simulink model "Differential_Equation"  (R2020b)
settings: Solver=VariableStepAuto  StartTime=0.0  StopTime=10.0  RelTol=1e-3
values from neighbouring files (symbols this model uses):
  a = 0.4    [data.mat]
  b = 0.5    [data.mat]
  c = 0.25    [data.mat]
settings Model: Creator=vijay jagtap  LastModifiedBy=vijay jagtap

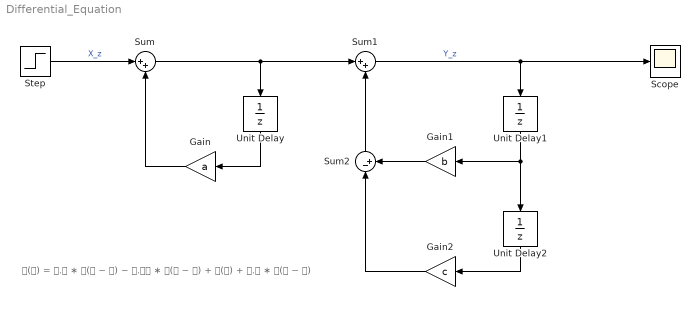
== system Differential_Equation ==
  note: 𝐲(𝐧) = 𝟎.𝟓 ∗ 𝐲(𝐧 − 𝟏) − 𝟎.𝟐𝟓 ∗ 𝐲(𝐧 − 𝟐) + 𝐱(𝐧) + 𝟎.𝟒 ∗ 𝐱(𝐧 − 𝟏)
  Gain : Gain  Gain=a
  Gain1 : Gain  Gain=b
  Gain2 : Gain  Gain=c
  Scope : Scope
  Step : Step  After=10  SampleTime=0
  Sum : Sum  Inputs=|++
  Sum1 : Sum  Inputs=|++
  Sum2 : Sum  Inputs=|-+
  Unit Delay : UnitDelay  SampleTime=-1  HasFrameUpgradeWarning=on
  Unit Delay1 : UnitDelay  SampleTime=-1  HasFrameUpgradeWarning=on
  Unit Delay2 : UnitDelay  SampleTime=-1  HasFrameUpgradeWarning=on
  wires:
  Sum2/1 -> Sum1/2
  Sum1/1 -> Scope/1, Unit Delay1/1  "Y_z"
  Gain1/1 -> Sum2/2
  Gain2/1 -> Sum2/1
  Unit Delay/1 -> Gain/1
  Gain/1 -> Sum/2
  Step/1 -> Sum/1  "X_z"
  Sum/1 -> Sum1/1, Unit Delay/1
  Unit Delay2/1 -> Gain2/1
  Unit Delay1/1 -> Gain1/1, Unit Delay2/1
